simulink model "arm_sim"  (R2016b)
settings: Solver=ode45  StartTime=0.0  StopTime=P.t_end  RelTol=1e-3  EnableMultiTasking=on
InitFcn:
  | addpath ./..
  | arm_param
  | armParamHW13
undefined symbols (not defined in the file or in its folder): arm_ctrl, P
settings Model: Creator=beard  LastModifiedBy=beard
settings DataIOCC: LimitDataPoints=on  SaveFormat=Array  SignalLoggingSaveFormat=ModelDataLogs
settings OptimizationCC: ExpressionDepthLimit=2147483647  InitFltsAndDblsToZero=on  LifeSpan=inf
settings DebuggingCC: UnderspecifiedInitializationDetection=Classic  MergeDetectMultiDrivingBlocksExec=none  SolverPrmCheckMsg=warning  FcnCallInpInsideContextMsg=warning  StateNameClashWarn=warning  SFUnexpectedBacktrackingDiag=warning  SFNoUnconditionalDefaultTransitionDiag=warning  SFExecutionAtInitializationDiag=none
settings HardwareCC: ProdBitPerPointer=32  ProdBitPerSizeT=32  ProdBitPerPtrDiffT=32  ProdLargestAtomicFloat=None  ProdIntDivRoundTo=Undefined  ProdEndianess=Unspecified  ProdWordSize=32  ProdHWDeviceType=32-bit Generic
settings ModelReferenceCC: PropagateSignalLabelsOutOfModel=off
settings GRTTargetCC: TargetLangStandard=C89/C90 (ANSI)  GeneratePreprocessorConditionals=Disable all  CombineOutputUpdateFcns=off  GRTInterface=on
settings ConfigComp: CovMetricSettings=dw  CovHtmlReporting=on  CovSaveCumulativeToWorkspaceVar=on  CovSaveSingleToWorkspaceVar=on  CovExternalEMLEnable=off

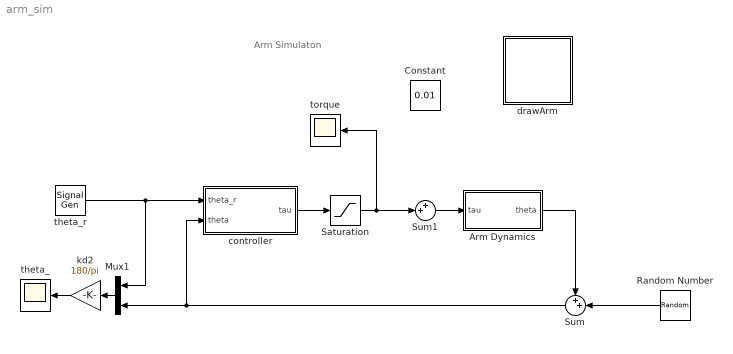
== system arm_sim ==
  note: Arm Simulaton
  "Arm Dynamics " : Subsystem
  Constant : Constant  Value=0.01
  Mux1 : Mux  Inputs=2
  Random Number : RandomNumber  Variance=.01^2  SampleTime=0.1
  Saturation : Saturate  UpperLimit=P.tau_max  LowerLimit=-P.tau_max
  Sum : Sum  Inputs=++|
  Sum1 : Sum  Inputs=++|
  controller : Subsystem
  drawArm : Subsystem
      mask Display: image(imread('tv.jpg'))
  kd2 : Gain  Gain=180/pi
  theta_ : Scope
  theta_r : SignalGenerator  WaveForm=square  Amplitude=25*pi/180  Frequency=.05
  torque : Scope
  wires:
  theta_r/1 -> controller/1(theta_r), Mux1/1
  Mux1/1 -> kd2/1
  kd2/1 -> theta_/1
  controller/1(tau) -> Saturation/1
  Saturation/1 -> Sum1/2, torque/1
  Sum1/1 -> "Arm Dynamics "/1(tau)
  "Arm Dynamics "/1("theta ") -> Sum/1
  Sum/1 -> controller/2(theta), Mux1/2
  Random Number/1 -> Sum/2

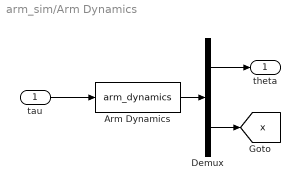
== system arm_sim/Arm Dynamics  ==
  tau : Inport
  Arm Dynamics : S-Function  FunctionName=arm_dynamics  Parameters=P  SFunctionDeploymentMode=off  EnableBusSupport=off
  Demux : Demux  Outputs=[1;2]
  "theta " : Outport
  tag scope: x=global
  wires:
  tau/1 -> Arm Dynamics/1
  Demux/1 -> "theta "/1
  Demux/2 -> [x]
  Arm Dynamics/1 -> Demux/1

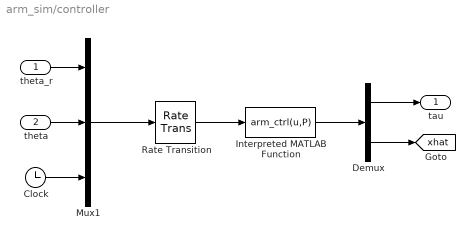
== system arm_sim/controller ==
  theta_r : Inport
  theta : Inport  Port=2
  Clock : Clock
  Demux : Demux  Outputs=[1;2]
  Interpreted MATLAB Function : MATLABFcn  MATLABFcn=arm_ctrl(u,P)  OutputDimensions=1+2
  Mux1 : Mux  Inputs=3
  Rate Transition : RateTransition  OutPortSampleTime=P.Ts
  tau : Outport
  tag scope: xhat=global
  wires:
  Demux/2 -> [xhat]
  Demux/1 -> tau/1
  Interpreted MATLAB Function/1 -> Demux/1
  Rate Transition/1 -> Interpreted MATLAB Function/1
  Clock/1 -> Mux1/3
  theta/1 -> Mux1/2
  theta_r/1 -> Mux1/1
  Mux1/1 -> Rate Transition/1

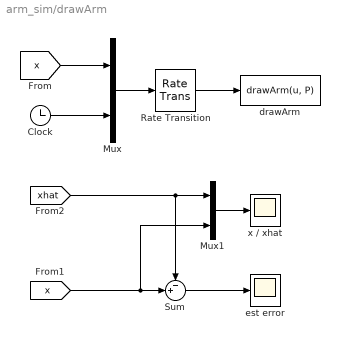
== system arm_sim/drawArm ==
  Clock : Clock
  Mux : Mux  Inputs=2
  Mux1 : Mux  Inputs=2
  Rate Transition : RateTransition  OutPortSampleTime=P.t_plot
  Sum : Sum  Inputs=-+|
  drawArm : MATLABFcn  MATLABFcn=drawArm(u, P)  OutputDimensions=0
  est error : Scope
  x / xhat : Scope
  wires:
  Rate Transition/1 -> drawArm/1
  Mux/1 -> Rate Transition/1
  Clock/1 -> Mux/2
  [x] -> Mux/1
  Mux1/1 -> x / xhat/1
  Sum/1 -> est error/1
  [xhat] -> Sum/1, Mux1/1
  [x] -> Sum/2, Mux1/2
